simulink model "dog_x_bit_true_2023_final"  (R2023a)
settings: Solver=ode45  StartTime=0.0  StopTime=1.5*lsim*Ts  MaxStep=1/f0/2  RelTol=1e-6
values from neighbouring files (symbols this model uses):
  ft = (bint-1)*fbin    [exe_DOG_X_bit_true_2023a.m]    (also in exe_DOG_X_integer_true_two_paths_5b.m)
  g1 = g1_ideal*1    (= 4)    [exe_DOG_X_bit_true_2023a.m]    (also in exe_DOG_X_integer_true_two_paths_5b.m)
  Kvco = f0    (= 99840000)    [exe_DOG_X_bit_true_2023a.m]    (also in exe_DOG_X_integer_true_two_paths_5b.m)
  lvl = Vfs*10^(Input_signal_dB/20)    (= 0.125892541179)    [exe_DOG_X_bit_true_2023a.m]    (also in exe_DOG_X_integer_true_two_paths_5b.m)
  Nbsv1 = Nbvco+4    (= 9)    [exe_DOG_X_bit_true_2023a.m]    (also in exe_DOG_X_integer_true_two_paths_5b.m)
  Nbsv2 = Nbsv1+Nbext    [exe_DOG_X_bit_true_2023a.m]    (also in exe_DOG_X_integer_true_two_paths_5b.m)
  pnoi = 10^(-(60)/10)*(Vfs^2/2)    (= 5e-07)    [exe_DOG_X_bit_true_2023a.m]    (also in exe_DOG_X_integer_true_two_paths_5b.m)
  T2 = 1/f2    (= 4.06901041667e-08)    [exe_DOG_X_bit_true_2023a.m]    (also in exe_DOG_X_integer_true_two_paths_5b.m)
  Ts = 1/fs    (= 3.25520833333e-07)    [exe_DOG_X_bit_true_2023a.m]    (also in exe_DOG_X_integer_true_two_paths_5b.m)
  Vfs = 1    [exe_DOG_X_bit_true_2023a.m]    (also in exe_DOG_X_integer_true_two_paths_5b.m)
undefined symbols (not defined in the file or in its folder): fa, fb
libraries: simulink_extras x86, simulink x7
(part 2 of 4)

== system dog_x_bit_true_2023_final/TOP/roX/vdly11 ==
  In : Inport
  C : Inport  Port=2
  Integrator : Integrator  InitialCondition=-1  LimitOutput=on  UpperSaturationLimit=1  LowerSaturationLimit=-1
  Product : Product  RndMeth=Zero
  Relay : Relay  OffOutputValue=-1
  Out : Outport  VectorParamsAs1DForOutWhenUnconnected=off
  wires:
  Relay/1 -> Out/1
  Product/1 -> Integrator/1
  Integrator/1 -> Relay/1
  C/1 -> Product/1
  In/1 -> Product/2

== system dog_x_bit_true_2023_final/TOP/roX/vdly12 ==
  In : Inport
  C : Inport  Port=2
  Integrator : Integrator  InitialCondition=-1  LimitOutput=on  UpperSaturationLimit=1  LowerSaturationLimit=-1
  Product : Product  RndMeth=Zero
  Relay : Relay  OffOutputValue=-1
  Out : Outport  VectorParamsAs1DForOutWhenUnconnected=off
  wires:
  Relay/1 -> Out/1
  Product/1 -> Integrator/1
  Integrator/1 -> Relay/1
  C/1 -> Product/1
  In/1 -> Product/2

== system dog_x_bit_true_2023_final/TOP/roX/vdly13 ==
  In : Inport
  C : Inport  Port=2
  Integrator : Integrator  InitialCondition=-1  LimitOutput=on  UpperSaturationLimit=1  LowerSaturationLimit=-1
  Product : Product  RndMeth=Zero
  Relay : Relay  OffOutputValue=-1
  Out : Outport  VectorParamsAs1DForOutWhenUnconnected=off
  wires:
  Relay/1 -> Out/1
  Product/1 -> Integrator/1
  Integrator/1 -> Relay/1
  C/1 -> Product/1
  In/1 -> Product/2

== system dog_x_bit_true_2023_final/TOP/roX/vdly14 ==
  In : Inport
  C : Inport  Port=2
  Integrator : Integrator  InitialCondition=-1  LimitOutput=on  UpperSaturationLimit=1  LowerSaturationLimit=-1
  Product : Product  RndMeth=Zero
  Relay : Relay  OffOutputValue=-1
  Out : Outport  VectorParamsAs1DForOutWhenUnconnected=off
  wires:
  Relay/1 -> Out/1
  Product/1 -> Integrator/1
  Integrator/1 -> Relay/1
  C/1 -> Product/1
  In/1 -> Product/2

== system dog_x_bit_true_2023_final/TOP/roX/vdly15 ==
  In : Inport
  C : Inport  Port=2
  Integrator : Integrator  InitialCondition=-1  LimitOutput=on  UpperSaturationLimit=1  LowerSaturationLimit=-1
  Product : Product  RndMeth=Zero
  Relay : Relay  OffOutputValue=-1
  Out : Outport  VectorParamsAs1DForOutWhenUnconnected=off
  wires:
  Relay/1 -> Out/1
  Product/1 -> Integrator/1
  Integrator/1 -> Relay/1
  C/1 -> Product/1
  In/1 -> Product/2

== system dog_x_bit_true_2023_final/TOP/roX/vdly16 ==
  In : Inport
  C : Inport  Port=2
  Integrator : Integrator  InitialCondition=-1  LimitOutput=on  UpperSaturationLimit=1  LowerSaturationLimit=-1
  Product : Product  RndMeth=Zero
  Relay : Relay  OffOutputValue=-1
  Out : Outport  VectorParamsAs1DForOutWhenUnconnected=off
  wires:
  Relay/1 -> Out/1
  Product/1 -> Integrator/1
  Integrator/1 -> Relay/1
  C/1 -> Product/1
  In/1 -> Product/2

== system dog_x_bit_true_2023_final/TOP/roX/vdly2 ==
  In : Inport
  C : Inport  Port=2
  Integrator : Integrator  InitialCondition=-1  LimitOutput=on  UpperSaturationLimit=1  LowerSaturationLimit=-1
  Product : Product  RndMeth=Zero
  Relay : Relay  OffOutputValue=-1
  Out : Outport  VectorParamsAs1DForOutWhenUnconnected=off
  wires:
  Relay/1 -> Out/1
  Product/1 -> Integrator/1
  Integrator/1 -> Relay/1
  C/1 -> Product/1
  In/1 -> Product/2

== system dog_x_bit_true_2023_final/TOP/roX/vdly3 ==
  In : Inport
  C : Inport  Port=2
  Integrator : Integrator  InitialCondition=-1  LimitOutput=on  UpperSaturationLimit=1  LowerSaturationLimit=-1
  Product : Product  RndMeth=Zero
  Relay : Relay  OffOutputValue=-1
  Out : Outport  VectorParamsAs1DForOutWhenUnconnected=off
  wires:
  Relay/1 -> Out/1
  Product/1 -> Integrator/1
  Integrator/1 -> Relay/1
  C/1 -> Product/1
  In/1 -> Product/2

== system dog_x_bit_true_2023_final/TOP/roX/vdly4 ==
  In : Inport
  C : Inport  Port=2
  Integrator : Integrator  InitialCondition=-1  LimitOutput=on  UpperSaturationLimit=1  LowerSaturationLimit=-1
  Product : Product  RndMeth=Zero
  Relay : Relay  OffOutputValue=-1
  Out : Outport  VectorParamsAs1DForOutWhenUnconnected=off
  wires:
  Relay/1 -> Out/1
  Product/1 -> Integrator/1
  Integrator/1 -> Relay/1
  C/1 -> Product/1
  In/1 -> Product/2

== system dog_x_bit_true_2023_final/TOP/roX/vdly5 ==
  In : Inport
  C : Inport  Port=2
  Integrator : Integrator  InitialCondition=-1  LimitOutput=on  UpperSaturationLimit=1  LowerSaturationLimit=-1
  Product : Product  RndMeth=Zero
  Relay : Relay  OffOutputValue=-1
  Out : Outport  VectorParamsAs1DForOutWhenUnconnected=off
  wires:
  Relay/1 -> Out/1
  Product/1 -> Integrator/1
  Integrator/1 -> Relay/1
  C/1 -> Product/1
  In/1 -> Product/2

== system dog_x_bit_true_2023_final/TOP/roX/vdly6 ==
  In : Inport
  C : Inport  Port=2
  Integrator : Integrator  InitialCondition=-1  LimitOutput=on  UpperSaturationLimit=1  LowerSaturationLimit=-1
  Product : Product  RndMeth=Zero
  Relay : Relay  OffOutputValue=-1
  Out : Outport  VectorParamsAs1DForOutWhenUnconnected=off
  wires:
  Relay/1 -> Out/1
  Product/1 -> Integrator/1
  Integrator/1 -> Relay/1
  C/1 -> Product/1
  In/1 -> Product/2

== system dog_x_bit_true_2023_final/TOP/roX/vdly7 ==
  In : Inport
  C : Inport  Port=2
  Integrator : Integrator  InitialCondition=-1  LimitOutput=on  UpperSaturationLimit=1  LowerSaturationLimit=-1
  Product : Product  RndMeth=Zero
  Relay : Relay  OffOutputValue=-1
  Out : Outport  VectorParamsAs1DForOutWhenUnconnected=off
  wires:
  Relay/1 -> Out/1
  Product/1 -> Integrator/1
  Integrator/1 -> Relay/1
  C/1 -> Product/1
  In/1 -> Product/2

== system dog_x_bit_true_2023_final/TOP/roX/vdly8 ==
  In : Inport
  C : Inport  Port=2
  Integrator : Integrator  InitialCondition=-1  LimitOutput=on  UpperSaturationLimit=1  LowerSaturationLimit=-1
  Product : Product  RndMeth=Zero
  Relay : Relay  OffOutputValue=-1
  Out : Outport  VectorParamsAs1DForOutWhenUnconnected=off
  wires:
  Relay/1 -> Out/1
  Product/1 -> Integrator/1
  Integrator/1 -> Relay/1
  C/1 -> Product/1
  In/1 -> Product/2

== system dog_x_bit_true_2023_final/TOP/roX/vdly9 ==
  In : Inport
  C : Inport  Port=2
  Integrator : Integrator  InitialCondition=-1  LimitOutput=on  UpperSaturationLimit=1  LowerSaturationLimit=-1
  Product : Product  RndMeth=Zero
  Relay : Relay  OffOutputValue=-1
  Out : Outport  VectorParamsAs1DForOutWhenUnconnected=off
  wires:
  Relay/1 -> Out/1
  Product/1 -> Integrator/1
  Integrator/1 -> Relay/1
  C/1 -> Product/1
  In/1 -> Product/2

== system dog_x_bit_true_2023_final/TOP/roX1/vdly1 ==
  In : Inport
  C : Inport  Port=2
  Integrator : Integrator  InitialCondition=-1  LimitOutput=on  UpperSaturationLimit=1  LowerSaturationLimit=-1
  Product : Product  RndMeth=Zero
  Relay : Relay  OffOutputValue=-1
  Out : Outport  VectorParamsAs1DForOutWhenUnconnected=off
  wires:
  Relay/1 -> Out/1
  Product/1 -> Integrator/1
  Integrator/1 -> Relay/1
  C/1 -> Product/1
  In/1 -> Product/2

== system dog_x_bit_true_2023_final/TOP/roX1/vdly10 ==
  In : Inport
  C : Inport  Port=2
  Integrator : Integrator  InitialCondition=-1  LimitOutput=on  UpperSaturationLimit=1  LowerSaturationLimit=-1
  Product : Product  RndMeth=Zero
  Relay : Relay  OffOutputValue=-1
  Out : Outport  VectorParamsAs1DForOutWhenUnconnected=off
  wires:
  Relay/1 -> Out/1
  Product/1 -> Integrator/1
  Integrator/1 -> Relay/1
  C/1 -> Product/1
  In/1 -> Product/2

== system dog_x_bit_true_2023_final/TOP/roX1/vdly11 ==
  In : Inport
  C : Inport  Port=2
  Integrator : Integrator  InitialCondition=-1  LimitOutput=on  UpperSaturationLimit=1  LowerSaturationLimit=-1
  Product : Product  RndMeth=Zero
  Relay : Relay  OffOutputValue=-1
  Out : Outport  VectorParamsAs1DForOutWhenUnconnected=off
  wires:
  Relay/1 -> Out/1
  Product/1 -> Integrator/1
  Integrator/1 -> Relay/1
  C/1 -> Product/1
  In/1 -> Product/2

== system dog_x_bit_true_2023_final/TOP/roX1/vdly12 ==
  In : Inport
  C : Inport  Port=2
  Integrator : Integrator  InitialCondition=-1  LimitOutput=on  UpperSaturationLimit=1  LowerSaturationLimit=-1
  Product : Product  RndMeth=Zero
  Relay : Relay  OffOutputValue=-1
  Out : Outport  VectorParamsAs1DForOutWhenUnconnected=off
  wires:
  Relay/1 -> Out/1
  Product/1 -> Integrator/1
  Integrator/1 -> Relay/1
  C/1 -> Product/1
  In/1 -> Product/2

== system dog_x_bit_true_2023_final/TOP/roX1/vdly13 ==
  In : Inport
  C : Inport  Port=2
  Integrator : Integrator  InitialCondition=-1  LimitOutput=on  UpperSaturationLimit=1  LowerSaturationLimit=-1
  Product : Product  RndMeth=Zero
  Relay : Relay  OffOutputValue=-1
  Out : Outport  VectorParamsAs1DForOutWhenUnconnected=off
  wires:
  Relay/1 -> Out/1
  Product/1 -> Integrator/1
  Integrator/1 -> Relay/1
  C/1 -> Product/1
  In/1 -> Product/2

== system dog_x_bit_true_2023_final/TOP/roX1/vdly14 ==
  In : Inport
  C : Inport  Port=2
  Integrator : Integrator  InitialCondition=-1  LimitOutput=on  UpperSaturationLimit=1  LowerSaturationLimit=-1
  Product : Product  RndMeth=Zero
  Relay : Relay  OffOutputValue=-1
  Out : Outport  VectorParamsAs1DForOutWhenUnconnected=off
  wires:
  Relay/1 -> Out/1
  Product/1 -> Integrator/1
  Integrator/1 -> Relay/1
  C/1 -> Product/1
  In/1 -> Product/2

== system dog_x_bit_true_2023_final/TOP/roX1/vdly15 ==
  In : Inport
  C : Inport  Port=2
  Integrator : Integrator  InitialCondition=-1  LimitOutput=on  UpperSaturationLimit=1  LowerSaturationLimit=-1
  Product : Product  RndMeth=Zero
  Relay : Relay  OffOutputValue=-1
  Out : Outport  VectorParamsAs1DForOutWhenUnconnected=off
  wires:
  Relay/1 -> Out/1
  Product/1 -> Integrator/1
  Integrator/1 -> Relay/1
  C/1 -> Product/1
  In/1 -> Product/2

== system dog_x_bit_true_2023_final/TOP/roX1/vdly16 ==
  In : Inport
  C : Inport  Port=2
  Integrator : Integrator  InitialCondition=-1  LimitOutput=on  UpperSaturationLimit=1  LowerSaturationLimit=-1
  Product : Product  RndMeth=Zero
  Relay : Relay  OffOutputValue=-1
  Out : Outport  VectorParamsAs1DForOutWhenUnconnected=off
  wires:
  Relay/1 -> Out/1
  Product/1 -> Integrator/1
  Integrator/1 -> Relay/1
  C/1 -> Product/1
  In/1 -> Product/2

== system dog_x_bit_true_2023_final/TOP/roX1/vdly2 ==
  In : Inport
  C : Inport  Port=2
  Integrator : Integrator  InitialCondition=-1  LimitOutput=on  UpperSaturationLimit=1  LowerSaturationLimit=-1
  Product : Product  RndMeth=Zero
  Relay : Relay  OffOutputValue=-1
  Out : Outport  VectorParamsAs1DForOutWhenUnconnected=off
  wires:
  Relay/1 -> Out/1
  Product/1 -> Integrator/1
  Integrator/1 -> Relay/1
  C/1 -> Product/1
  In/1 -> Product/2

== system dog_x_bit_true_2023_final/TOP/roX1/vdly3 ==
  In : Inport
  C : Inport  Port=2
  Integrator : Integrator  InitialCondition=-1  LimitOutput=on  UpperSaturationLimit=1  LowerSaturationLimit=-1
  Product : Product  RndMeth=Zero
  Relay : Relay  OffOutputValue=-1
  Out : Outport  VectorParamsAs1DForOutWhenUnconnected=off
  wires:
  Relay/1 -> Out/1
  Product/1 -> Integrator/1
  Integrator/1 -> Relay/1
  C/1 -> Product/1
  In/1 -> Product/2

== system dog_x_bit_true_2023_final/TOP/roX1/vdly4 ==
  In : Inport
  C : Inport  Port=2
  Integrator : Integrator  InitialCondition=-1  LimitOutput=on  UpperSaturationLimit=1  LowerSaturationLimit=-1
  Product : Product  RndMeth=Zero
  Relay : Relay  OffOutputValue=-1
  Out : Outport  VectorParamsAs1DForOutWhenUnconnected=off
  wires:
  Relay/1 -> Out/1
  Product/1 -> Integrator/1
  Integrator/1 -> Relay/1
  C/1 -> Product/1
  In/1 -> Product/2

== system dog_x_bit_true_2023_final/TOP/roX1/vdly5 ==
  In : Inport
  C : Inport  Port=2
  Integrator : Integrator  InitialCondition=-1  LimitOutput=on  UpperSaturationLimit=1  LowerSaturationLimit=-1
  Product : Product  RndMeth=Zero
  Relay : Relay  OffOutputValue=-1
  Out : Outport  VectorParamsAs1DForOutWhenUnconnected=off
  wires:
  Relay/1 -> Out/1
  Product/1 -> Integrator/1
  Integrator/1 -> Relay/1
  C/1 -> Product/1
  In/1 -> Product/2

== system dog_x_bit_true_2023_final/TOP/roX1/vdly6 ==
  In : Inport
  C : Inport  Port=2
  Integrator : Integrator  InitialCondition=-1  LimitOutput=on  UpperSaturationLimit=1  LowerSaturationLimit=-1
  Product : Product  RndMeth=Zero
  Relay : Relay  OffOutputValue=-1
  Out : Outport  VectorParamsAs1DForOutWhenUnconnected=off
  wires:
  Relay/1 -> Out/1
  Product/1 -> Integrator/1
  Integrator/1 -> Relay/1
  C/1 -> Product/1
  In/1 -> Product/2

== system dog_x_bit_true_2023_final/TOP/roX1/vdly7 ==
  In : Inport
  C : Inport  Port=2
  Integrator : Integrator  InitialCondition=-1  LimitOutput=on  UpperSaturationLimit=1  LowerSaturationLimit=-1
  Product : Product  RndMeth=Zero
  Relay : Relay  OffOutputValue=-1
  Out : Outport  VectorParamsAs1DForOutWhenUnconnected=off
  wires:
  Relay/1 -> Out/1
  Product/1 -> Integrator/1
  Integrator/1 -> Relay/1
  C/1 -> Product/1
  In/1 -> Product/2

== system dog_x_bit_true_2023_final/TOP/roX1/vdly8 ==
  In : Inport
  C : Inport  Port=2
  Integrator : Integrator  InitialCondition=-1  LimitOutput=on  UpperSaturationLimit=1  LowerSaturationLimit=-1
  Product : Product  RndMeth=Zero
  Relay : Relay  OffOutputValue=-1
  Out : Outport  VectorParamsAs1DForOutWhenUnconnected=off
  wires:
  Relay/1 -> Out/1
  Product/1 -> Integrator/1
  Integrator/1 -> Relay/1
  C/1 -> Product/1
  In/1 -> Product/2

== system dog_x_bit_true_2023_final/TOP/roX1/vdly9 ==
  In : Inport
  C : Inport  Port=2
  Integrator : Integrator  InitialCondition=-1  LimitOutput=on  UpperSaturationLimit=1  LowerSaturationLimit=-1
  Product : Product  RndMeth=Zero
  Relay : Relay  OffOutputValue=-1
  Out : Outport  VectorParamsAs1DForOutWhenUnconnected=off
  wires:
  Relay/1 -> Out/1
  Product/1 -> Integrator/1
  Integrator/1 -> Relay/1
  C/1 -> Product/1
  In/1 -> Product/2

== system dog_x_bit_true_2023_final/TOP/roX2/vdly1 ==
  In : Inport
  C : Inport  Port=2
  Integrator : Integrator  InitialCondition=-1  LimitOutput=on  UpperSaturationLimit=1  LowerSaturationLimit=-1
  Product : Product  RndMeth=Zero
  Relay : Relay  OffOutputValue=-1
  Out : Outport  VectorParamsAs1DForOutWhenUnconnected=off
  wires:
  Relay/1 -> Out/1
  Product/1 -> Integrator/1
  Integrator/1 -> Relay/1
  C/1 -> Product/1
  In/1 -> Product/2

== system dog_x_bit_true_2023_final/TOP/roX2/vdly10 ==
  In : Inport
  C : Inport  Port=2
  Integrator : Integrator  InitialCondition=-1  LimitOutput=on  UpperSaturationLimit=1  LowerSaturationLimit=-1
  Product : Product  RndMeth=Zero
  Relay : Relay  OffOutputValue=-1
  Out : Outport  VectorParamsAs1DForOutWhenUnconnected=off
  wires:
  Relay/1 -> Out/1
  Product/1 -> Integrator/1
  Integrator/1 -> Relay/1
  C/1 -> Product/1
  In/1 -> Product/2

== system dog_x_bit_true_2023_final/TOP/roX2/vdly11 ==
  In : Inport
  C : Inport  Port=2
  Integrator : Integrator  InitialCondition=-1  LimitOutput=on  UpperSaturationLimit=1  LowerSaturationLimit=-1
  Product : Product  RndMeth=Zero
  Relay : Relay  OffOutputValue=-1
  Out : Outport  VectorParamsAs1DForOutWhenUnconnected=off
  wires:
  Relay/1 -> Out/1
  Product/1 -> Integrator/1
  Integrator/1 -> Relay/1
  C/1 -> Product/1
  In/1 -> Product/2

== system dog_x_bit_true_2023_final/TOP/roX2/vdly12 ==
  In : Inport
  C : Inport  Port=2
  Integrator : Integrator  InitialCondition=-1  LimitOutput=on  UpperSaturationLimit=1  LowerSaturationLimit=-1
  Product : Product  RndMeth=Zero
  Relay : Relay  OffOutputValue=-1
  Out : Outport  VectorParamsAs1DForOutWhenUnconnected=off
  wires:
  Relay/1 -> Out/1
  Product/1 -> Integrator/1
  Integrator/1 -> Relay/1
  C/1 -> Product/1
  In/1 -> Product/2

== system dog_x_bit_true_2023_final/TOP/roX2/vdly13 ==
  In : Inport
  C : Inport  Port=2
  Integrator : Integrator  InitialCondition=-1  LimitOutput=on  UpperSaturationLimit=1  LowerSaturationLimit=-1
  Product : Product  RndMeth=Zero
  Relay : Relay  OffOutputValue=-1
  Out : Outport  VectorParamsAs1DForOutWhenUnconnected=off
  wires:
  Relay/1 -> Out/1
  Product/1 -> Integrator/1
  Integrator/1 -> Relay/1
  C/1 -> Product/1
  In/1 -> Product/2

== system dog_x_bit_true_2023_final/TOP/roX2/vdly14 ==
  In : Inport
  C : Inport  Port=2
  Integrator : Integrator  InitialCondition=-1  LimitOutput=on  UpperSaturationLimit=1  LowerSaturationLimit=-1
  Product : Product  RndMeth=Zero
  Relay : Relay  OffOutputValue=-1
  Out : Outport  VectorParamsAs1DForOutWhenUnconnected=off
  wires:
  Relay/1 -> Out/1
  Product/1 -> Integrator/1
  Integrator/1 -> Relay/1
  C/1 -> Product/1
  In/1 -> Product/2

== system dog_x_bit_true_2023_final/TOP/roX2/vdly15 ==
  In : Inport
  C : Inport  Port=2
  Integrator : Integrator  InitialCondition=-1  LimitOutput=on  UpperSaturationLimit=1  LowerSaturationLimit=-1
  Product : Product  RndMeth=Zero
  Relay : Relay  OffOutputValue=-1
  Out : Outport  VectorParamsAs1DForOutWhenUnconnected=off
  wires:
  Relay/1 -> Out/1
  Product/1 -> Integrator/1
  Integrator/1 -> Relay/1
  C/1 -> Product/1
  In/1 -> Product/2

== system dog_x_bit_true_2023_final/TOP/roX2/vdly16 ==
  In : Inport
  C : Inport  Port=2
  Integrator : Integrator  InitialCondition=-1  LimitOutput=on  UpperSaturationLimit=1  LowerSaturationLimit=-1
  Product : Product  RndMeth=Zero
  Relay : Relay  OffOutputValue=-1
  Out : Outport  VectorParamsAs1DForOutWhenUnconnected=off
  wires:
  Relay/1 -> Out/1
  Product/1 -> Integrator/1
  Integrator/1 -> Relay/1
  C/1 -> Product/1
  In/1 -> Product/2

== system dog_x_bit_true_2023_final/TOP/roX2/vdly2 ==
  In : Inport
  C : Inport  Port=2
  Integrator : Integrator  InitialCondition=-1  LimitOutput=on  UpperSaturationLimit=1  LowerSaturationLimit=-1
  Product : Product  RndMeth=Zero
  Relay : Relay  OffOutputValue=-1
  Out : Outport  VectorParamsAs1DForOutWhenUnconnected=off
  wires:
  Relay/1 -> Out/1
  Product/1 -> Integrator/1
  Integrator/1 -> Relay/1
  C/1 -> Product/1
  In/1 -> Product/2

== system dog_x_bit_true_2023_final/TOP/roX2/vdly3 ==
  In : Inport
  C : Inport  Port=2
  Integrator : Integrator  InitialCondition=-1  LimitOutput=on  UpperSaturationLimit=1  LowerSaturationLimit=-1
  Product : Product  RndMeth=Zero
  Relay : Relay  OffOutputValue=-1
  Out : Outport  VectorParamsAs1DForOutWhenUnconnected=off
  wires:
  Relay/1 -> Out/1
  Product/1 -> Integrator/1
  Integrator/1 -> Relay/1
  C/1 -> Product/1
  In/1 -> Product/2

== system dog_x_bit_true_2023_final/TOP/roX2/vdly4 ==
  In : Inport
  C : Inport  Port=2
  Integrator : Integrator  InitialCondition=-1  LimitOutput=on  UpperSaturationLimit=1  LowerSaturationLimit=-1
  Product : Product  RndMeth=Zero
  Relay : Relay  OffOutputValue=-1
  Out : Outport  VectorParamsAs1DForOutWhenUnconnected=off
  wires:
  Relay/1 -> Out/1
  Product/1 -> Integrator/1
  Integrator/1 -> Relay/1
  C/1 -> Product/1
  In/1 -> Product/2

== system dog_x_bit_true_2023_final/TOP/roX2/vdly5 ==
  In : Inport
  C : Inport  Port=2
  Integrator : Integrator  InitialCondition=-1  LimitOutput=on  UpperSaturationLimit=1  LowerSaturationLimit=-1
  Product : Product  RndMeth=Zero
  Relay : Relay  OffOutputValue=-1
  Out : Outport  VectorParamsAs1DForOutWhenUnconnected=off
  wires:
  Relay/1 -> Out/1
  Product/1 -> Integrator/1
  Integrator/1 -> Relay/1
  C/1 -> Product/1
  In/1 -> Product/2

== system dog_x_bit_true_2023_final/TOP/roX2/vdly6 ==
  In : Inport
  C : Inport  Port=2
  Integrator : Integrator  InitialCondition=-1  LimitOutput=on  UpperSaturationLimit=1  LowerSaturationLimit=-1
  Product : Product  RndMeth=Zero
  Relay : Relay  OffOutputValue=-1
  Out : Outport  VectorParamsAs1DForOutWhenUnconnected=off
  wires:
  Relay/1 -> Out/1
  Product/1 -> Integrator/1
  Integrator/1 -> Relay/1
  C/1 -> Product/1
  In/1 -> Product/2

== system dog_x_bit_true_2023_final/TOP/roX2/vdly7 ==
  In : Inport
  C : Inport  Port=2
  Integrator : Integrator  InitialCondition=-1  LimitOutput=on  UpperSaturationLimit=1  LowerSaturationLimit=-1
  Product : Product  RndMeth=Zero
  Relay : Relay  OffOutputValue=-1
  Out : Outport  VectorParamsAs1DForOutWhenUnconnected=off
  wires:
  Relay/1 -> Out/1
  Product/1 -> Integrator/1
  Integrator/1 -> Relay/1
  C/1 -> Product/1
  In/1 -> Product/2

== system dog_x_bit_true_2023_final/TOP/roX2/vdly8 ==
  In : Inport
  C : Inport  Port=2
  Integrator : Integrator  InitialCondition=-1  LimitOutput=on  UpperSaturationLimit=1  LowerSaturationLimit=-1
  Product : Product  RndMeth=Zero
  Relay : Relay  OffOutputValue=-1
  Out : Outport  VectorParamsAs1DForOutWhenUnconnected=off
  wires:
  Relay/1 -> Out/1
  Product/1 -> Integrator/1
  Integrator/1 -> Relay/1
  C/1 -> Product/1
  In/1 -> Product/2

== system dog_x_bit_true_2023_final/TOP/roX2/vdly9 ==
  In : Inport
  C : Inport  Port=2
  Integrator : Integrator  InitialCondition=-1  LimitOutput=on  UpperSaturationLimit=1  LowerSaturationLimit=-1
  Product : Product  RndMeth=Zero
  Relay : Relay  OffOutputValue=-1
  Out : Outport  VectorParamsAs1DForOutWhenUnconnected=off
  wires:
  Relay/1 -> Out/1
  Product/1 -> Integrator/1
  Integrator/1 -> Relay/1
  C/1 -> Product/1
  In/1 -> Product/2

== system dog_x_bit_true_2023_final/TOP/roX3/vdly1 ==
  In : Inport
  C : Inport  Port=2
  Integrator : Integrator  InitialCondition=-1  LimitOutput=on  UpperSaturationLimit=1  LowerSaturationLimit=-1
  Product : Product  RndMeth=Zero
  Relay : Relay  OffOutputValue=-1
  Out : Outport  VectorParamsAs1DForOutWhenUnconnected=off
  wires:
  Relay/1 -> Out/1
  Product/1 -> Integrator/1
  Integrator/1 -> Relay/1
  C/1 -> Product/1
  In/1 -> Product/2

== system dog_x_bit_true_2023_final/TOP/roX3/vdly10 ==
  In : Inport
  C : Inport  Port=2
  Integrator : Integrator  InitialCondition=-1  LimitOutput=on  UpperSaturationLimit=1  LowerSaturationLimit=-1
  Product : Product  RndMeth=Zero
  Relay : Relay  OffOutputValue=-1
  Out : Outport  VectorParamsAs1DForOutWhenUnconnected=off
  wires:
  Relay/1 -> Out/1
  Product/1 -> Integrator/1
  Integrator/1 -> Relay/1
  C/1 -> Product/1
  In/1 -> Product/2

== system dog_x_bit_true_2023_final/TOP/roX3/vdly11 ==
  In : Inport
  C : Inport  Port=2
  Integrator : Integrator  InitialCondition=-1  LimitOutput=on  UpperSaturationLimit=1  LowerSaturationLimit=-1
  Product : Product  RndMeth=Zero
  Relay : Relay  OffOutputValue=-1
  Out : Outport  VectorParamsAs1DForOutWhenUnconnected=off
  wires:
  Relay/1 -> Out/1
  Product/1 -> Integrator/1
  Integrator/1 -> Relay/1
  C/1 -> Product/1
  In/1 -> Product/2

== system dog_x_bit_true_2023_final/TOP/roX3/vdly12 ==
  In : Inport
  C : Inport  Port=2
  Integrator : Integrator  InitialCondition=-1  LimitOutput=on  UpperSaturationLimit=1  LowerSaturationLimit=-1
  Product : Product  RndMeth=Zero
  Relay : Relay  OffOutputValue=-1
  Out : Outport  VectorParamsAs1DForOutWhenUnconnected=off
  wires:
  Relay/1 -> Out/1
  Product/1 -> Integrator/1
  Integrator/1 -> Relay/1
  C/1 -> Product/1
  In/1 -> Product/2

== system dog_x_bit_true_2023_final/TOP/roX3/vdly13 ==
  In : Inport
  C : Inport  Port=2
  Integrator : Integrator  InitialCondition=-1  LimitOutput=on  UpperSaturationLimit=1  LowerSaturationLimit=-1
  Product : Product  RndMeth=Zero
  Relay : Relay  OffOutputValue=-1
  Out : Outport  VectorParamsAs1DForOutWhenUnconnected=off
  wires:
  Relay/1 -> Out/1
  Product/1 -> Integrator/1
  Integrator/1 -> Relay/1
  C/1 -> Product/1
  In/1 -> Product/2

== system dog_x_bit_true_2023_final/TOP/roX3/vdly14 ==
  In : Inport
  C : Inport  Port=2
  Integrator : Integrator  InitialCondition=-1  LimitOutput=on  UpperSaturationLimit=1  LowerSaturationLimit=-1
  Product : Product  RndMeth=Zero
  Relay : Relay  OffOutputValue=-1
  Out : Outport  VectorParamsAs1DForOutWhenUnconnected=off
  wires:
  Relay/1 -> Out/1
  Product/1 -> Integrator/1
  Integrator/1 -> Relay/1
  C/1 -> Product/1
  In/1 -> Product/2

== system dog_x_bit_true_2023_final/TOP/roX3/vdly15 ==
  In : Inport
  C : Inport  Port=2
  Integrator : Integrator  InitialCondition=-1  LimitOutput=on  UpperSaturationLimit=1  LowerSaturationLimit=-1
  Product : Product  RndMeth=Zero
  Relay : Relay  OffOutputValue=-1
  Out : Outport  VectorParamsAs1DForOutWhenUnconnected=off
  wires:
  Relay/1 -> Out/1
  Product/1 -> Integrator/1
  Integrator/1 -> Relay/1
  C/1 -> Product/1
  In/1 -> Product/2

== system dog_x_bit_true_2023_final/TOP/roX3/vdly16 ==
  In : Inport
  C : Inport  Port=2
  Integrator : Integrator  InitialCondition=-1  LimitOutput=on  UpperSaturationLimit=1  LowerSaturationLimit=-1
  Product : Product  RndMeth=Zero
  Relay : Relay  OffOutputValue=-1
  Out : Outport  VectorParamsAs1DForOutWhenUnconnected=off
  wires:
  Relay/1 -> Out/1
  Product/1 -> Integrator/1
  Integrator/1 -> Relay/1
  C/1 -> Product/1
  In/1 -> Product/2

== system dog_x_bit_true_2023_final/TOP/roX3/vdly2 ==
  In : Inport
  C : Inport  Port=2
  Integrator : Integrator  InitialCondition=-1  LimitOutput=on  UpperSaturationLimit=1  LowerSaturationLimit=-1
  Product : Product  RndMeth=Zero
  Relay : Relay  OffOutputValue=-1
  Out : Outport  VectorParamsAs1DForOutWhenUnconnected=off
  wires:
  Relay/1 -> Out/1
  Product/1 -> Integrator/1
  Integrator/1 -> Relay/1
  C/1 -> Product/1
  In/1 -> Product/2

== system dog_x_bit_true_2023_final/TOP/roX3/vdly3 ==
  In : Inport
  C : Inport  Port=2
  Integrator : Integrator  InitialCondition=-1  LimitOutput=on  UpperSaturationLimit=1  LowerSaturationLimit=-1
  Product : Product  RndMeth=Zero
  Relay : Relay  OffOutputValue=-1
  Out : Outport  VectorParamsAs1DForOutWhenUnconnected=off
  wires:
  Relay/1 -> Out/1
  Product/1 -> Integrator/1
  Integrator/1 -> Relay/1
  C/1 -> Product/1
  In/1 -> Product/2

== system dog_x_bit_true_2023_final/TOP/roX3/vdly4 ==
  In : Inport
  C : Inport  Port=2
  Integrator : Integrator  InitialCondition=-1  LimitOutput=on  UpperSaturationLimit=1  LowerSaturationLimit=-1
  Product : Product  RndMeth=Zero
  Relay : Relay  OffOutputValue=-1
  Out : Outport  VectorParamsAs1DForOutWhenUnconnected=off
  wires:
  Relay/1 -> Out/1
  Product/1 -> Integrator/1
  Integrator/1 -> Relay/1
  C/1 -> Product/1
  In/1 -> Product/2

== system dog_x_bit_true_2023_final/TOP/roX3/vdly5 ==
  In : Inport
  C : Inport  Port=2
  Integrator : Integrator  InitialCondition=-1  LimitOutput=on  UpperSaturationLimit=1  LowerSaturationLimit=-1
  Product : Product  RndMeth=Zero
  Relay : Relay  OffOutputValue=-1
  Out : Outport  VectorParamsAs1DForOutWhenUnconnected=off
  wires:
  Relay/1 -> Out/1
  Product/1 -> Integrator/1
  Integrator/1 -> Relay/1
  C/1 -> Product/1
  In/1 -> Product/2

== system dog_x_bit_true_2023_final/TOP/roX3/vdly6 ==
  In : Inport
  C : Inport  Port=2
  Integrator : Integrator  InitialCondition=-1  LimitOutput=on  UpperSaturationLimit=1  LowerSaturationLimit=-1
  Product : Product  RndMeth=Zero
  Relay : Relay  OffOutputValue=-1
  Out : Outport  VectorParamsAs1DForOutWhenUnconnected=off
  wires:
  Relay/1 -> Out/1
  Product/1 -> Integrator/1
  Integrator/1 -> Relay/1
  C/1 -> Product/1
  In/1 -> Product/2

== system dog_x_bit_true_2023_final/TOP/roX3/vdly7 ==
  In : Inport
  C : Inport  Port=2
  Integrator : Integrator  InitialCondition=-1  LimitOutput=on  UpperSaturationLimit=1  LowerSaturationLimit=-1
  Product : Product  RndMeth=Zero
  Relay : Relay  OffOutputValue=-1
  Out : Outport  VectorParamsAs1DForOutWhenUnconnected=off
  wires:
  Relay/1 -> Out/1
  Product/1 -> Integrator/1
  Integrator/1 -> Relay/1
  C/1 -> Product/1
  In/1 -> Product/2

== system dog_x_bit_true_2023_final/TOP/roX3/vdly8 ==
  In : Inport
  C : Inport  Port=2
  Integrator : Integrator  InitialCondition=-1  LimitOutput=on  UpperSaturationLimit=1  LowerSaturationLimit=-1
  Product : Product  RndMeth=Zero
  Relay : Relay  OffOutputValue=-1
  Out : Outport  VectorParamsAs1DForOutWhenUnconnected=off
  wires:
  Relay/1 -> Out/1
  Product/1 -> Integrator/1
  Integrator/1 -> Relay/1
  C/1 -> Product/1
  In/1 -> Product/2

== system dog_x_bit_true_2023_final/TOP/roX3/vdly9 ==
  In : Inport
  C : Inport  Port=2
  Integrator : Integrator  InitialCondition=-1  LimitOutput=on  UpperSaturationLimit=1  LowerSaturationLimit=-1
  Product : Product  RndMeth=Zero
  Relay : Relay  OffOutputValue=-1
  Out : Outport  VectorParamsAs1DForOutWhenUnconnected=off
  wires:
  Relay/1 -> Out/1
  Product/1 -> Integrator/1
  Integrator/1 -> Relay/1
  C/1 -> Product/1
  In/1 -> Product/2

== system dog_x_bit_true_2023_final/TOP/Subsystem/Noise_shaper_HDR/ 2 bit arithmetic right shift ==
  in : Inport
  Demux1 : Demux  Outputs=11
  Mux : Mux  Inputs=9
  Terminator1 : Terminator
  Terminator3 : Terminator
  9 MSB : Outport
  wires:
  Mux/1 -> 9 MSB/1
  in/1 -> Demux1/1
  Demux1/11 -> Terminator1/1
  Demux1/10 -> Terminator3/1
  Demux1/1 -> Mux/1
  Demux1/2 -> Mux/2
  Demux1/3 -> Mux/3
  Demux1/4 -> Mux/4
  Demux1/5 -> Mux/5
  Demux1/6 -> Mux/6
  Demux1/7 -> Mux/7
  Demux1/8 -> Mux/8
  Demux1/9 -> Mux/9

== system dog_x_bit_true_2023_final/TOP/Subsystem/Noise_shaper_HDR/DCO ==
  clock : Inport
  control : Inport  Port=2
  accumulator (11 bits) : Subsystem
  register1 : Subsystem
  output : Outport
  wires:
  clock/1 -> register1/1(CLK)
  control/1 -> accumulator (11 bits)/1(plus)
  accumulator (11 bits)/1(subs) -> register1/2(D)
  register1/1(Q) -> output/1, accumulator (11 bits)/2(feedback)

== system dog_x_bit_true_2023_final/TOP/Subsystem/Noise_shaper_HDR/differential substraction (9 bit) ==
  counter P : Inport
  conter N : Inport  Port=2
  Constant : Constant  OutDataTypeStr=boolean
  Demux : Demux  Outputs=9
  Demux1 : Demux  Outputs=9
  FA : Subsystem
  FA1 : Subsystem
  FA2 : Subsystem
  FA3 : Subsystem
  FA4 : Subsystem
  FA5 : Subsystem
  FA6 : Subsystem
  FA7 : Subsystem
  FA8 : Subsystem
  Mux : Mux  Inputs=9
  NOT : Logic  Operator=NOT  IconShape=distinctive  AllPortsSameDT=off  OutDataTypeStr=boolean
  Terminator2 : Terminator
  subs : Outport
  wires:
  Mux/1 -> subs/1
  counter P/1 -> Demux/1
  conter N/1 -> NOT/1
  NOT/1 -> Demux1/1
  FA7/2(Co) -> FA6/3(Cin)
  FA6/2(Co) -> FA5/3(Cin)
  FA5/2(Co) -> FA4/3(Cin)
  FA4/2(Co) -> FA3/3(Cin)
  FA3/2(Co) -> FA2/3(Cin)
  FA2/2(Co) -> FA1/3(Cin)
  FA1/2(Co) -> FA/3(Cin)
  FA/2(Co) -> FA8/3(Cin)
  FA8/2(Co) -> Terminator2/1
  FA8/1(S) -> Mux/1
  FA/1(S) -> Mux/2
  FA1/1(S) -> Mux/3
  FA2/1(S) -> Mux/4
  FA3/1(S) -> Mux/5
  FA4/1(S) -> Mux/6
  FA5/1(S) -> Mux/7
  FA6/1(S) -> Mux/8
  FA7/1(S) -> Mux/9
  Demux/1 -> FA8/1(B0)
  Demux/2 -> FA/1(B0)
  Demux/3 -> FA1/1(B0)
  Demux/4 -> FA2/1(B0)
  Demux/5 -> FA3/1(B0)
  Demux/6 -> FA4/1(B0)
  Demux/7 -> FA5/1(B0)
  Demux/8 -> FA6/1(B0)
  Demux/9 -> FA7/1(B0)
  Demux1/9 -> FA7/2(B1)
  Demux1/8 -> FA6/2(B1)
  Demux1/7 -> FA5/2(B1)
  Demux1/6 -> FA4/2(B1)
  Demux1/5 -> FA3/2(B1)
  Demux1/4 -> FA2/2(B1)
  Demux1/3 -> FA1/2(B1)
  Demux1/2 -> FA/2(B1)
  Demux1/1 -> FA8/2(B1)
  Constant/1 -> FA7/3(Cin)

== system dog_x_bit_true_2023_final/TOP/Subsystem/Noise_shaper_HDR/feedback substraction (9 bit) ==
  plus : Inport
  minus : Inport  Port=2
  Constant : Constant  OutDataTypeStr=boolean
  Demux : Demux  Outputs=9
  Demux1 : Demux  Outputs=9
  FA : Subsystem
  FA1 : Subsystem
  FA2 : Subsystem
  FA3 : Subsystem
  FA4 : Subsystem
  FA5 : Subsystem
  FA6 : Subsystem
  FA7 : Subsystem
  FA8 : Subsystem
  Mux : Mux  Inputs=9
  NOT : Logic  Operator=NOT  IconShape=distinctive  AllPortsSameDT=off  OutDataTypeStr=boolean
  Terminator2 : Terminator
  subs : Outport
  wires:
  Mux/1 -> subs/1
  plus/1 -> Demux/1
  minus/1 -> NOT/1
  NOT/1 -> Demux1/1
  FA7/2(Co) -> FA6/3(Cin)
  FA6/2(Co) -> FA5/3(Cin)
  FA5/2(Co) -> FA4/3(Cin)
  FA4/2(Co) -> FA3/3(Cin)
  FA3/2(Co) -> FA2/3(Cin)
  FA2/2(Co) -> FA1/3(Cin)
  FA1/2(Co) -> FA/3(Cin)
  FA/2(Co) -> FA8/3(Cin)
  FA8/2(Co) -> Terminator2/1
  FA8/1(S) -> Mux/1
  FA/1(S) -> Mux/2
  FA1/1(S) -> Mux/3
  FA2/1(S) -> Mux/4
  FA3/1(S) -> Mux/5
  FA4/1(S) -> Mux/6
  FA5/1(S) -> Mux/7
  FA6/1(S) -> Mux/8
  FA7/1(S) -> Mux/9
  Demux/1 -> FA8/1(B0)
  Demux/2 -> FA/1(B0)
  Demux/3 -> FA1/1(B0)
  Demux/4 -> FA2/1(B0)
  Demux/5 -> FA3/1(B0)
  Demux/6 -> FA4/1(B0)
  Demux/7 -> FA5/1(B0)
  Demux/8 -> FA6/1(B0)
  Demux/9 -> FA7/1(B0)
  Demux1/9 -> FA7/2(B1)
  Demux1/8 -> FA6/2(B1)
  Demux1/7 -> FA5/2(B1)
  Demux1/6 -> FA4/2(B1)
  Demux1/5 -> FA3/2(B1)
  Demux1/4 -> FA2/2(B1)
  Demux1/3 -> FA1/2(B1)
  Demux1/2 -> FA/2(B1)
  Demux1/1 -> FA8/2(B1)
  Constant/1 -> FA7/3(Cin)

== system dog_x_bit_true_2023_final/TOP/Subsystem/Noise_shaper_HDR/first difference substraction (9 bit) ==
  plus : Inport
  minus : Inport  Port=2
  Constant : Constant  OutDataTypeStr=boolean
  Demux : Demux  Outputs=9
  Demux1 : Demux  Outputs=9
  FA : Subsystem
  FA1 : Subsystem
  FA2 : Subsystem
  FA3 : Subsystem
  FA4 : Subsystem
  FA5 : Subsystem
  FA6 : Subsystem
  FA7 : Subsystem
  FA8 : Subsystem
  Mux : Mux  Inputs=9
  NOT : Logic  Operator=NOT  IconShape=distinctive  AllPortsSameDT=off  OutDataTypeStr=boolean
  Terminator2 : Terminator
  subs : Outport
  wires:
  Mux/1 -> subs/1
  plus/1 -> Demux/1
  minus/1 -> NOT/1
  NOT/1 -> Demux1/1
  FA7/2(Co) -> FA6/3(Cin)
  FA6/2(Co) -> FA5/3(Cin)
  FA5/2(Co) -> FA4/3(Cin)
  FA4/2(Co) -> FA3/3(Cin)
  FA3/2(Co) -> FA2/3(Cin)
  FA2/2(Co) -> FA1/3(Cin)
  FA1/2(Co) -> FA/3(Cin)
  FA/2(Co) -> FA8/3(Cin)
  FA8/2(Co) -> Terminator2/1
  FA8/1(S) -> Mux/1
  FA/1(S) -> Mux/2
  FA1/1(S) -> Mux/3
  FA2/1(S) -> Mux/4
  FA3/1(S) -> Mux/5
  FA4/1(S) -> Mux/6
  FA5/1(S) -> Mux/7
  FA6/1(S) -> Mux/8
  FA7/1(S) -> Mux/9
  Demux/1 -> FA8/1(B0)
  Demux/2 -> FA/1(B0)
  Demux/3 -> FA1/1(B0)
  Demux/4 -> FA2/1(B0)
  Demux/5 -> FA3/1(B0)
  Demux/6 -> FA4/1(B0)
  Demux/7 -> FA5/1(B0)
  Demux/8 -> FA6/1(B0)
  Demux/9 -> FA7/1(B0)
  Demux1/9 -> FA7/2(B1)
  Demux1/8 -> FA6/2(B1)
  Demux1/7 -> FA5/2(B1)
  Demux1/6 -> FA4/2(B1)
  Demux1/5 -> FA3/2(B1)
  Demux1/4 -> FA2/2(B1)
  Demux1/3 -> FA1/2(B1)
  Demux1/2 -> FA/2(B1)
  Demux1/1 -> FA8/2(B1)
  Constant/1 -> FA7/3(Cin)

== system dog_x_bit_true_2023_final/TOP/Subsystem/Noise_shaper_HDR/first difference substraction (9 bit)2 ==
  plus : Inport
  minus : Inport  Port=2
  Constant : Constant  OutDataTypeStr=boolean
  Demux : Demux  Outputs=9
  Demux1 : Demux  Outputs=9
  FA : Subsystem
  FA1 : Subsystem
  FA2 : Subsystem
  FA3 : Subsystem
  FA4 : Subsystem
  FA5 : Subsystem
  FA6 : Subsystem
  FA7 : Subsystem
  FA8 : Subsystem
  Mux : Mux  Inputs=9
  NOT : Logic  Operator=NOT  IconShape=distinctive  AllPortsSameDT=off  OutDataTypeStr=boolean
  Terminator2 : Terminator
  subs : Outport
  wires:
  Mux/1 -> subs/1
  plus/1 -> Demux/1
  minus/1 -> NOT/1
  NOT/1 -> Demux1/1
  FA7/2(Co) -> FA6/3(Cin)
  FA6/2(Co) -> FA5/3(Cin)
  FA5/2(Co) -> FA4/3(Cin)
  FA4/2(Co) -> FA3/3(Cin)
  FA3/2(Co) -> FA2/3(Cin)
  FA2/2(Co) -> FA1/3(Cin)
  FA1/2(Co) -> FA/3(Cin)
  FA/2(Co) -> FA8/3(Cin)
  FA8/2(Co) -> Terminator2/1
  FA8/1(S) -> Mux/1
  FA/1(S) -> Mux/2
  FA1/1(S) -> Mux/3
  FA2/1(S) -> Mux/4
  FA3/1(S) -> Mux/5
  FA4/1(S) -> Mux/6
  FA5/1(S) -> Mux/7
  FA6/1(S) -> Mux/8
  FA7/1(S) -> Mux/9
  Demux/1 -> FA8/1(B0)
  Demux/2 -> FA/1(B0)
  Demux/3 -> FA1/1(B0)
  Demux/4 -> FA2/1(B0)
  Demux/5 -> FA3/1(B0)
  Demux/6 -> FA4/1(B0)
  Demux/7 -> FA5/1(B0)
  Demux/8 -> FA6/1(B0)
  Demux/9 -> FA7/1(B0)
  Demux1/9 -> FA7/2(B1)
  Demux1/8 -> FA6/2(B1)
  Demux1/7 -> FA5/2(B1)
  Demux1/6 -> FA4/2(B1)
  Demux1/5 -> FA3/2(B1)
  Demux1/4 -> FA2/2(B1)
  Demux1/3 -> FA1/2(B1)
  Demux1/2 -> FA/2(B1)
  Demux1/1 -> FA8/2(B1)
  Constant/1 -> FA7/3(Cin)

== system dog_x_bit_true_2023_final/TOP/Subsystem/Noise_shaper_HDR/offset correction ==
  a : Inport
  b : Inport  Port=2
  Constant : Constant  Value=0  OutDataTypeStr=boolean
  Demux : Demux  Outputs=9
  Demux1 : Demux
  FA : Subsystem
  FA1 : Subsystem
  FA2 : Subsystem
  FA3 : Subsystem
  FA4 : Subsystem
  FA5 : Subsystem
  FA6 : Subsystem
  FA7 : Subsystem
  FA8 : Subsystem
  Mux : Mux  Inputs=9
  Terminator2 : Terminator
  sum : Outport
  wires:
  Mux/1 -> sum/1
  b/1 -> Demux1/1
  FA7/2(Co) -> FA6/3(Cin)
  FA6/2(Co) -> FA5/3(Cin)
  FA5/2(Co) -> FA4/3(Cin)
  FA4/2(Co) -> FA3/3(Cin)
  FA3/2(Co) -> FA2/3(Cin)
  FA2/2(Co) -> FA1/3(Cin)
  FA1/2(Co) -> FA/3(Cin)
  FA/2(Co) -> FA8/3(Cin)
  FA8/2(Co) -> Terminator2/1
  FA8/1(S) -> Mux/1
  FA/1(S) -> Mux/2
  FA1/1(S) -> Mux/3
  FA2/1(S) -> Mux/4
  FA3/1(S) -> Mux/5
  FA4/1(S) -> Mux/6
  FA5/1(S) -> Mux/7
  FA6/1(S) -> Mux/8
  FA7/1(S) -> Mux/9
  Demux/1 -> FA8/1(B0)
  Demux/2 -> FA/1(B0)
  Demux/3 -> FA1/1(B0)
  Demux/4 -> FA2/1(B0)
  Demux/5 -> FA3/1(B0)
  Demux/6 -> FA4/1(B0)
  Demux/7 -> FA5/1(B0)
  Demux/8 -> FA6/1(B0)
  Demux/9 -> FA7/1(B0)
  Constant/1 -> FA7/3(Cin)
  Demux1/4 -> FA7/2(B1)
  Demux1/3 -> FA6/2(B1)
  Demux1/2 -> FA5/2(B1)
  Demux1/1 -> FA3/2(B1), FA2/2(B1), FA1/2(B1), FA/2(B1), FA8/2(B1), FA4/2(B1)
  a/1 -> Demux/1

== system dog_x_bit_true_2023_final/TOP/Subsystem/Noise_shaper_HDR/register2 ==
  CLK : Inport
  D : Inport  Port=2
  Constant4 : Constant  OutDataTypeStr=boolean
  D Flip-Flop : simulink_extras/Flip Flops/D Flip-Flop
  Terminator : Terminator
  Q : Outport
  wires:
  Constant4/1 -> D Flip-Flop/3
  CLK/1 -> D Flip-Flop/2
  D Flip-Flop/2 -> Terminator/1
  D Flip-Flop/1 -> Q/1
  D/1 -> D Flip-Flop/1

== system dog_x_bit_true_2023_final/TOP/Subsystem/Noise_shaper_HDR/register3 ==
  CLK : Inport
  D : Inport  Port=2
  Constant4 : Constant  OutDataTypeStr=boolean
  D Flip-Flop : simulink_extras/Flip Flops/D Flip-Flop
  Terminator : Terminator
  Q : Outport
  wires:
  Constant4/1 -> D Flip-Flop/3
  CLK/1 -> D Flip-Flop/2
  D Flip-Flop/2 -> Terminator/1
  D Flip-Flop/1 -> Q/1
  D/1 -> D Flip-Flop/1

== system dog_x_bit_true_2023_final/TOP/Subsystem/Noise_shaper_HDR/register4 ==
  CLK : Inport
  D : Inport  Port=2
  Constant4 : Constant  OutDataTypeStr=boolean
  D Flip-Flop : simulink_extras/Flip Flops/D Flip-Flop
  Terminator : Terminator
  Q : Outport
  wires:
  Constant4/1 -> D Flip-Flop/3
  CLK/1 -> D Flip-Flop/2
  D Flip-Flop/2 -> Terminator/1
  D Flip-Flop/1 -> Q/1
  D/1 -> D Flip-Flop/1

== system dog_x_bit_true_2023_final/TOP/Subsystem/Noise_shaper_HDR/register5 ==
  CLK : Inport
  D : Inport  Port=2
  Constant4 : Constant  OutDataTypeStr=boolean
  D Flip-Flop : simulink_extras/Flip Flops/D Flip-Flop
  Terminator : Terminator
  Q : Outport
  wires:
  Constant4/1 -> D Flip-Flop/3
  CLK/1 -> D Flip-Flop/2
  D Flip-Flop/2 -> Terminator/1
  D Flip-Flop/1 -> Q/1
  D/1 -> D Flip-Flop/1

== system dog_x_bit_true_2023_final/TOP/Subsystem/Noise_shaper_HSNR/ 2 bit arithmetic right shift ==
  in : Inport
  Demux1 : Demux  Outputs=11
  Mux : Mux  Inputs=9
  Terminator1 : Terminator
  Terminator3 : Terminator
  9 MSB : Outport
  wires:
  Mux/1 -> 9 MSB/1
  in/1 -> Demux1/1
  Demux1/11 -> Terminator1/1
  Demux1/10 -> Terminator3/1
  Demux1/1 -> Mux/1
  Demux1/2 -> Mux/2
  Demux1/3 -> Mux/3
  Demux1/4 -> Mux/4
  Demux1/5 -> Mux/5
  Demux1/6 -> Mux/6
  Demux1/7 -> Mux/7
  Demux1/8 -> Mux/8
  Demux1/9 -> Mux/9

== system dog_x_bit_true_2023_final/TOP/Subsystem/Noise_shaper_HSNR/DCO ==
  clock : Inport
  control : Inport  Port=2
  accumulator (11 bits) : Subsystem
  register1 : Subsystem
  output : Outport
  wires:
  clock/1 -> register1/1(CLK)
  control/1 -> accumulator (11 bits)/1(plus)
  accumulator (11 bits)/1(subs) -> register1/2(D)
  register1/1(Q) -> output/1, accumulator (11 bits)/2(feedback)

== system dog_x_bit_true_2023_final/TOP/Subsystem/Noise_shaper_HSNR/differential substraction (9 bit) ==
  counter P : Inport
  conter N : Inport  Port=2
  Constant : Constant  OutDataTypeStr=boolean
  Demux : Demux  Outputs=9
  Demux1 : Demux  Outputs=9
  FA : Subsystem
  FA1 : Subsystem
  FA2 : Subsystem
  FA3 : Subsystem
  FA4 : Subsystem
  FA5 : Subsystem
  FA6 : Subsystem
  FA7 : Subsystem
  FA8 : Subsystem
  Mux : Mux  Inputs=9
  NOT : Logic  Operator=NOT  IconShape=distinctive  AllPortsSameDT=off  OutDataTypeStr=boolean
  Terminator2 : Terminator
  subs : Outport
  wires:
  Mux/1 -> subs/1
  counter P/1 -> Demux/1
  conter N/1 -> NOT/1
  NOT/1 -> Demux1/1
  FA7/2(Co) -> FA6/3(Cin)
  FA6/2(Co) -> FA5/3(Cin)
  FA5/2(Co) -> FA4/3(Cin)
  FA4/2(Co) -> FA3/3(Cin)
  FA3/2(Co) -> FA2/3(Cin)
  FA2/2(Co) -> FA1/3(Cin)
  FA1/2(Co) -> FA/3(Cin)
  FA/2(Co) -> FA8/3(Cin)
  FA8/2(Co) -> Terminator2/1
  FA8/1(S) -> Mux/1
  FA/1(S) -> Mux/2
  FA1/1(S) -> Mux/3
  FA2/1(S) -> Mux/4
  FA3/1(S) -> Mux/5
  FA4/1(S) -> Mux/6
  FA5/1(S) -> Mux/7
  FA6/1(S) -> Mux/8
  FA7/1(S) -> Mux/9
  Demux/1 -> FA8/1(B0)
  Demux/2 -> FA/1(B0)
  Demux/3 -> FA1/1(B0)
  Demux/4 -> FA2/1(B0)
  Demux/5 -> FA3/1(B0)
  Demux/6 -> FA4/1(B0)
  Demux/7 -> FA5/1(B0)
  Demux/8 -> FA6/1(B0)
  Demux/9 -> FA7/1(B0)
  Demux1/9 -> FA7/2(B1)
  Demux1/8 -> FA6/2(B1)
  Demux1/7 -> FA5/2(B1)
  Demux1/6 -> FA4/2(B1)
  Demux1/5 -> FA3/2(B1)
  Demux1/4 -> FA2/2(B1)
  Demux1/3 -> FA1/2(B1)
  Demux1/2 -> FA/2(B1)
  Demux1/1 -> FA8/2(B1)
  Constant/1 -> FA7/3(Cin)

== system dog_x_bit_true_2023_final/TOP/Subsystem/Noise_shaper_HSNR/feedback substraction (9 bit) ==
  plus : Inport
  minus : Inport  Port=2
  Constant : Constant  OutDataTypeStr=boolean
  Demux : Demux  Outputs=9
  Demux1 : Demux  Outputs=9
  FA : Subsystem
  FA1 : Subsystem
  FA2 : Subsystem
  FA3 : Subsystem
  FA4 : Subsystem
  FA5 : Subsystem
  FA6 : Subsystem
  FA7 : Subsystem
  FA8 : Subsystem
  Mux : Mux  Inputs=9
  NOT : Logic  Operator=NOT  IconShape=distinctive  AllPortsSameDT=off  OutDataTypeStr=boolean
  Terminator2 : Terminator
  subs : Outport
  wires:
  Mux/1 -> subs/1
  plus/1 -> Demux/1
  minus/1 -> NOT/1
  NOT/1 -> Demux1/1
  FA7/2(Co) -> FA6/3(Cin)
  FA6/2(Co) -> FA5/3(Cin)
  FA5/2(Co) -> FA4/3(Cin)
  FA4/2(Co) -> FA3/3(Cin)
  FA3/2(Co) -> FA2/3(Cin)
  FA2/2(Co) -> FA1/3(Cin)
  FA1/2(Co) -> FA/3(Cin)
  FA/2(Co) -> FA8/3(Cin)
  FA8/2(Co) -> Terminator2/1
  FA8/1(S) -> Mux/1
  FA/1(S) -> Mux/2
  FA1/1(S) -> Mux/3
  FA2/1(S) -> Mux/4
  FA3/1(S) -> Mux/5
  FA4/1(S) -> Mux/6
  FA5/1(S) -> Mux/7
  FA6/1(S) -> Mux/8
  FA7/1(S) -> Mux/9
  Demux/1 -> FA8/1(B0)
  Demux/2 -> FA/1(B0)
  Demux/3 -> FA1/1(B0)
  Demux/4 -> FA2/1(B0)
  Demux/5 -> FA3/1(B0)
  Demux/6 -> FA4/1(B0)
  Demux/7 -> FA5/1(B0)
  Demux/8 -> FA6/1(B0)
  Demux/9 -> FA7/1(B0)
  Demux1/9 -> FA7/2(B1)
  Demux1/8 -> FA6/2(B1)
  Demux1/7 -> FA5/2(B1)
  Demux1/6 -> FA4/2(B1)
  Demux1/5 -> FA3/2(B1)
  Demux1/4 -> FA2/2(B1)
  Demux1/3 -> FA1/2(B1)
  Demux1/2 -> FA/2(B1)
  Demux1/1 -> FA8/2(B1)
  Constant/1 -> FA7/3(Cin)

== system dog_x_bit_true_2023_final/TOP/Subsystem/Noise_shaper_HSNR/first difference substraction (9 bit) ==
  plus : Inport
  minus : Inport  Port=2
  Constant : Constant  OutDataTypeStr=boolean
  Demux : Demux  Outputs=9
  Demux1 : Demux  Outputs=9
  FA : Subsystem
  FA1 : Subsystem
  FA2 : Subsystem
  FA3 : Subsystem
  FA4 : Subsystem
  FA5 : Subsystem
  FA6 : Subsystem
  FA7 : Subsystem
  FA8 : Subsystem
  Mux : Mux  Inputs=9
  NOT : Logic  Operator=NOT  IconShape=distinctive  AllPortsSameDT=off  OutDataTypeStr=boolean
  Terminator2 : Terminator
  subs : Outport
  wires:
  Mux/1 -> subs/1
  plus/1 -> Demux/1
  minus/1 -> NOT/1
  NOT/1 -> Demux1/1
  FA7/2(Co) -> FA6/3(Cin)
  FA6/2(Co) -> FA5/3(Cin)
  FA5/2(Co) -> FA4/3(Cin)
  FA4/2(Co) -> FA3/3(Cin)
  FA3/2(Co) -> FA2/3(Cin)
  FA2/2(Co) -> FA1/3(Cin)
  FA1/2(Co) -> FA/3(Cin)
  FA/2(Co) -> FA8/3(Cin)
  FA8/2(Co) -> Terminator2/1
  FA8/1(S) -> Mux/1
  FA/1(S) -> Mux/2
  FA1/1(S) -> Mux/3
  FA2/1(S) -> Mux/4
  FA3/1(S) -> Mux/5
  FA4/1(S) -> Mux/6
  FA5/1(S) -> Mux/7
  FA6/1(S) -> Mux/8
  FA7/1(S) -> Mux/9
  Demux/1 -> FA8/1(B0)
  Demux/2 -> FA/1(B0)
  Demux/3 -> FA1/1(B0)
  Demux/4 -> FA2/1(B0)
  Demux/5 -> FA3/1(B0)
  Demux/6 -> FA4/1(B0)
  Demux/7 -> FA5/1(B0)
  Demux/8 -> FA6/1(B0)
  Demux/9 -> FA7/1(B0)
  Demux1/9 -> FA7/2(B1)
  Demux1/8 -> FA6/2(B1)
  Demux1/7 -> FA5/2(B1)
  Demux1/6 -> FA4/2(B1)
  Demux1/5 -> FA3/2(B1)
  Demux1/4 -> FA2/2(B1)
  Demux1/3 -> FA1/2(B1)
  Demux1/2 -> FA/2(B1)
  Demux1/1 -> FA8/2(B1)
  Constant/1 -> FA7/3(Cin)

== system dog_x_bit_true_2023_final/TOP/Subsystem/Noise_shaper_HSNR/first difference substraction (9 bit)2 ==
  plus : Inport
  minus : Inport  Port=2
  Constant : Constant  OutDataTypeStr=boolean
  Demux : Demux  Outputs=9
  Demux1 : Demux  Outputs=9
  FA : Subsystem
  FA1 : Subsystem
  FA2 : Subsystem
  FA3 : Subsystem
  FA4 : Subsystem
  FA5 : Subsystem
  FA6 : Subsystem
  FA7 : Subsystem
  FA8 : Subsystem
  Mux : Mux  Inputs=9
  NOT : Logic  Operator=NOT  IconShape=distinctive  AllPortsSameDT=off  OutDataTypeStr=boolean
  Terminator2 : Terminator
  subs : Outport
  wires:
  Mux/1 -> subs/1
  plus/1 -> Demux/1
  minus/1 -> NOT/1
  NOT/1 -> Demux1/1
  FA7/2(Co) -> FA6/3(Cin)
  FA6/2(Co) -> FA5/3(Cin)
  FA5/2(Co) -> FA4/3(Cin)
  FA4/2(Co) -> FA3/3(Cin)
  FA3/2(Co) -> FA2/3(Cin)
  FA2/2(Co) -> FA1/3(Cin)
  FA1/2(Co) -> FA/3(Cin)
  FA/2(Co) -> FA8/3(Cin)
  FA8/2(Co) -> Terminator2/1
  FA8/1(S) -> Mux/1
  FA/1(S) -> Mux/2
  FA1/1(S) -> Mux/3
  FA2/1(S) -> Mux/4
  FA3/1(S) -> Mux/5
  FA4/1(S) -> Mux/6
  FA5/1(S) -> Mux/7
  FA6/1(S) -> Mux/8
  FA7/1(S) -> Mux/9
  Demux/1 -> FA8/1(B0)
  Demux/2 -> FA/1(B0)
  Demux/3 -> FA1/1(B0)
  Demux/4 -> FA2/1(B0)
  Demux/5 -> FA3/1(B0)
  Demux/6 -> FA4/1(B0)
  Demux/7 -> FA5/1(B0)
  Demux/8 -> FA6/1(B0)
  Demux/9 -> FA7/1(B0)
  Demux1/9 -> FA7/2(B1)
  Demux1/8 -> FA6/2(B1)
  Demux1/7 -> FA5/2(B1)
  Demux1/6 -> FA4/2(B1)
  Demux1/5 -> FA3/2(B1)
  Demux1/4 -> FA2/2(B1)
  Demux1/3 -> FA1/2(B1)
  Demux1/2 -> FA/2(B1)
  Demux1/1 -> FA8/2(B1)
  Constant/1 -> FA7/3(Cin)

== system dog_x_bit_true_2023_final/TOP/Subsystem/Noise_shaper_HSNR/offset correction1 ==
  a : Inport
  b : Inport  Port=2
  Constant : Constant  Value=0  OutDataTypeStr=boolean
  Demux : Demux  Outputs=9
  Demux1 : Demux
  FA : Subsystem
  FA1 : Subsystem
  FA2 : Subsystem
  FA3 : Subsystem
  FA4 : Subsystem
  FA5 : Subsystem
  FA6 : Subsystem
  FA7 : Subsystem
  FA8 : Subsystem
  Mux : Mux  Inputs=9
  Terminator2 : Terminator
  sum : Outport
  wires:
  Mux/1 -> sum/1
  b/1 -> Demux1/1
  FA7/2(Co) -> FA6/3(Cin)
  FA6/2(Co) -> FA5/3(Cin)
  FA5/2(Co) -> FA4/3(Cin)
  FA4/2(Co) -> FA3/3(Cin)
  FA3/2(Co) -> FA2/3(Cin)
  FA2/2(Co) -> FA1/3(Cin)
  FA1/2(Co) -> FA/3(Cin)
  FA/2(Co) -> FA8/3(Cin)
  FA8/2(Co) -> Terminator2/1
  FA8/1(S) -> Mux/1
  FA/1(S) -> Mux/2
  FA1/1(S) -> Mux/3
  FA2/1(S) -> Mux/4
  FA3/1(S) -> Mux/5
  FA4/1(S) -> Mux/6
  FA5/1(S) -> Mux/7
  FA6/1(S) -> Mux/8
  FA7/1(S) -> Mux/9
  Demux/1 -> FA8/1(B0)
  Demux/2 -> FA/1(B0)
  Demux/3 -> FA1/1(B0)
  Demux/4 -> FA2/1(B0)
  Demux/5 -> FA3/1(B0)
  Demux/6 -> FA4/1(B0)
  Demux/7 -> FA5/1(B0)
  Demux/8 -> FA6/1(B0)
  Demux/9 -> FA7/1(B0)
  Constant/1 -> FA7/3(Cin)
  Demux1/4 -> FA7/2(B1)
  Demux1/3 -> FA6/2(B1)
  Demux1/2 -> FA5/2(B1)
  Demux1/1 -> FA3/2(B1), FA2/2(B1), FA1/2(B1), FA/2(B1), FA8/2(B1), FA4/2(B1)
  a/1 -> Demux/1

== system dog_x_bit_true_2023_final/TOP/Subsystem/Noise_shaper_HSNR/register2 ==
  CLK : Inport
  D : Inport  Port=2
  Constant4 : Constant  OutDataTypeStr=boolean
  D Flip-Flop : simulink_extras/Flip Flops/D Flip-Flop
  Terminator : Terminator
  Q : Outport
  wires:
  Constant4/1 -> D Flip-Flop/3
  CLK/1 -> D Flip-Flop/2
  D Flip-Flop/2 -> Terminator/1
  D Flip-Flop/1 -> Q/1
  D/1 -> D Flip-Flop/1

== system dog_x_bit_true_2023_final/TOP/Subsystem/Noise_shaper_HSNR/register3 ==
  CLK : Inport
  D : Inport  Port=2
  Constant4 : Constant  OutDataTypeStr=boolean
  D Flip-Flop : simulink_extras/Flip Flops/D Flip-Flop
  Terminator : Terminator
  Q : Outport
  wires:
  Constant4/1 -> D Flip-Flop/3
  CLK/1 -> D Flip-Flop/2
  D Flip-Flop/2 -> Terminator/1
  D Flip-Flop/1 -> Q/1
  D/1 -> D Flip-Flop/1

== system dog_x_bit_true_2023_final/TOP/Subsystem/Noise_shaper_HSNR/register4 ==
  CLK : Inport
  D : Inport  Port=2
  Constant4 : Constant  OutDataTypeStr=boolean
  D Flip-Flop : simulink_extras/Flip Flops/D Flip-Flop
  Terminator : Terminator
  Q : Outport
  wires:
  Constant4/1 -> D Flip-Flop/3
  CLK/1 -> D Flip-Flop/2
  D Flip-Flop/2 -> Terminator/1
  D Flip-Flop/1 -> Q/1
  D/1 -> D Flip-Flop/1

== system dog_x_bit_true_2023_final/TOP/Subsystem/Noise_shaper_HSNR/register5 ==
  CLK : Inport
  D : Inport  Port=2
  Constant4 : Constant  OutDataTypeStr=boolean
  D Flip-Flop : simulink_extras/Flip Flops/D Flip-Flop
  Terminator : Terminator
  Q : Outport
  wires:
  Constant4/1 -> D Flip-Flop/3
  CLK/1 -> D Flip-Flop/2
  D Flip-Flop/2 -> Terminator/1
  D Flip-Flop/1 -> Q/1
  D/1 -> D Flip-Flop/1

== system dog_x_bit_true_2023_final/TOP/Subsystem/progressive_mux/Subsystem ==
  select : Inport
  A : Inport  Port=2
  B : Inport  Port=3
  AND : Logic  IconShape=distinctive  AllPortsSameDT=off  OutDataTypeStr=boolean
  AND1 : Logic  IconShape=distinctive  AllPortsSameDT=off  OutDataTypeStr=boolean
  NOT : Logic  Operator=NOT  IconShape=distinctive  AllPortsSameDT=off  OutDataTypeStr=boolean
  OR : Logic  Operator=OR  IconShape=distinctive  AllPortsSameDT=off  OutDataTypeStr=boolean
  Y : Outport
  wires:
  AND/1 -> OR/1
  A/1 -> AND/1
  AND1/1 -> OR/2
  B/1 -> AND1/2
  select/1 -> NOT/1, AND/2
  NOT/1 -> AND1/1
  OR/1 -> Y/1
